simulink library "lib_Convection_SquareRodCrossFlowHilpert"  (R2015a)
settings: Solver=ode45  StartTime=0.0  StopTime=10.0  RelTol=1e-3
libraries: simulink x6
settings Model: Creator=jlkratz  LastModifiedBy=jlkratz

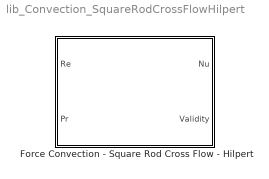
== system lib_Convection_SquareRodCrossFlowHilpert ==
  Force Convection - Square Rod Cross Flow - Hilpert : Subsystem  mask(TSAT: Square Rod Cross Flow - Hilpert){PointOrFace_M=Flow directed at a point of the square}
      mask help:
      | This block estimates the average Nusselt number of an external flow over an isothermal rod with a square cross-section. The correlation employed was originally developed by Hilpert and has been modified to address non-circular cross-sectional shapes. It has options to address the case in which the flow is directed at a point of the square or a side. Note that when the flow is directed at a face, the Reynolds number should be calculated based on the length of the sides of the square and when the flow is directed at a point, the Reynolds number should be calculated based on the length from opposite points of the square. The properties of the fluid should be evaluated at the film temperature. The correlation is subject to the following restrictions:
      |
      | Flow directed at a point of the square:
      | 6000 <= Re <= 60000
      | Pr >= 0.7
      |
      | Flow directed at a side of the square:
      | 5000 <= Re <= 60000
      | Pr >= 0.7
      |
      | For more information see the block help menu.
      mask Help: web(which('Convection_TSAT_SquareRodCrossFlowHilpert.html'),'-helpbrowser')
      mask TypeOptions PointOrFace_M: Flow directed at a point of the square | Flow directed at a side of the square

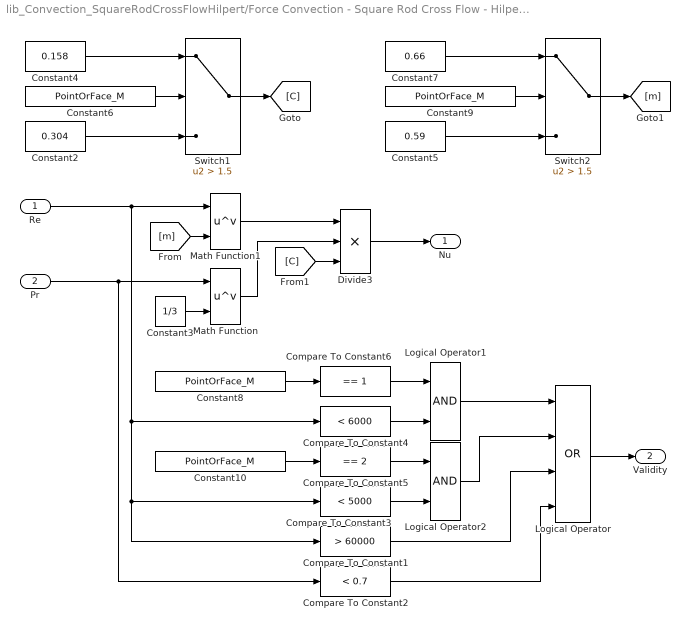
== system lib_Convection_SquareRodCrossFlowHilpert/Force Convection - Square Rod Cross Flow - Hilpert ==
  Re : Inport
  Pr : Inport  Port=2
  Compare To Constant1 : simulink/Logic and Bit Operations/Compare To Constant  relop=>  const=60000  OutDataTypeStr=boolean
  Compare To Constant2 : simulink/Logic and Bit Operations/Compare To Constant  relop=<  const=0.7  OutDataTypeStr=boolean
  Compare To Constant3 : simulink/Logic and Bit Operations/Compare To Constant  relop=<  const=5000  OutDataTypeStr=boolean
  Compare To Constant4 : simulink/Logic and Bit Operations/Compare To Constant  relop=<  const=6000  OutDataTypeStr=boolean
  Compare To Constant5 : simulink/Logic and Bit Operations/Compare To Constant  relop===  const=2  OutDataTypeStr=boolean
  Compare To Constant6 : simulink/Logic and Bit Operations/Compare To Constant  relop===  const=1  OutDataTypeStr=boolean
  Constant{6,8..10} (4 alike) : Constant  Value=PointOrFace_M
  Constant2 : Constant  Value=0.304
  Constant3 : Constant  Value=1/3
  Constant4 : Constant  Value=0.158
  Constant5 : Constant  Value=0.59
  Constant7 : Constant  Value=0.66
  Divide3 : Product  Inputs=***
  Logical Operator : Logic  Operator=OR  Inputs=4  AllPortsSameDT=off  OutDataTypeStr=boolean
  Logical Operator1 : Logic  AllPortsSameDT=off  OutDataTypeStr=boolean
  Logical Operator2 : Logic  AllPortsSameDT=off  OutDataTypeStr=boolean
  Math Function : Math  Operator=pow  SaturateOnIntegerOverflow=on
  Math Function1 : Math  Operator=pow  SaturateOnIntegerOverflow=on
  Switch1 : Switch  Criteria=u2 > Threshold  Threshold=1.5
  Switch2 : Switch  Criteria=u2 > Threshold  Threshold=1.5
  Nu : Outport
  Validity : Outport  Port=2
  wires:
  Logical Operator/1 -> Validity/1
  Compare To Constant1/1 -> Logical Operator/3
  Compare To Constant2/1 -> Logical Operator/4
  Logical Operator2/1 -> Logical Operator/2
  Logical Operator1/1 -> Logical Operator/1
  Compare To Constant3/1 -> Logical Operator2/2
  Compare To Constant5/1 -> Logical Operator2/1
  Compare To Constant4/1 -> Logical Operator1/2
  Compare To Constant6/1 -> Logical Operator1/1
  Constant10/1 -> Compare To Constant5/1
  Constant8/1 -> Compare To Constant6/1
  [C] -> Divide3/3
  Switch2/1 -> [m]
  Constant9/1 -> Switch2/2
  Constant7/1 -> Switch2/1
  Constant5/1 -> Switch2/3
  Switch1/1 -> [C]
  Constant6/1 -> Switch1/2
  Constant4/1 -> Switch1/1
  Constant2/1 -> Switch1/3
  Divide3/1 -> Nu/1
  Math Function1/1 -> Divide3/1
  Pr/1 -> Math Function/1, Compare To Constant2/1
  Re/1 -> Math Function1/1, Compare To Constant4/1, Compare To Constant3/1, Compare To Constant1/1
  [m] -> Math Function1/2
  Constant3/1 -> Math Function/2
  Math Function/1 -> Divide3/2
